simulink model "Task1_d"  (R2024b)
settings: Solver=VariableStepAuto  StartTime=0.0  StopTime=10.0  RelTol=1e-3
settings Model: Creator=max  LastModifiedBy=max

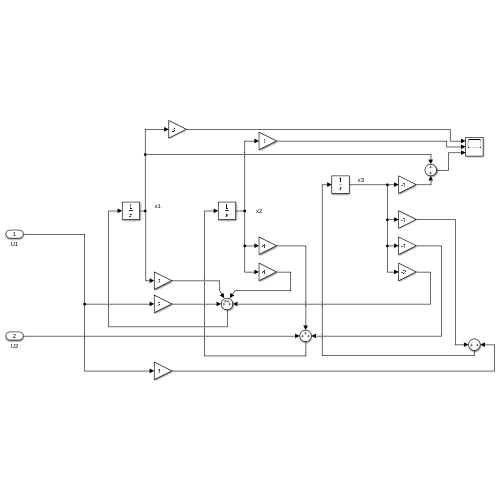
[thumbnail: Simulink's stored preview of the top-level diagram]
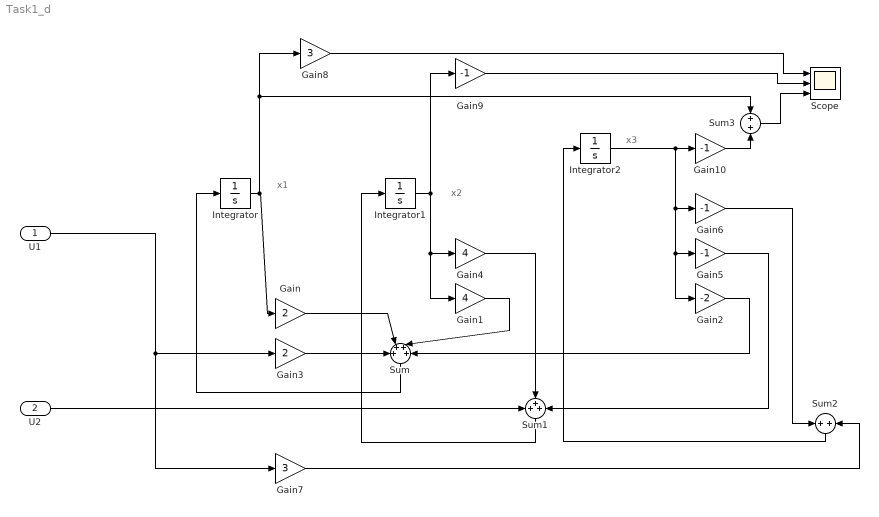
== system Task1_d ==
  note: x1
  note: x2
  note: x3
  U1 : Inport
  U2 : Inport  Port=2
  Gain : Gain  Gain=2
  Gain1 : Gain  Gain=4
  Gain{5..6,9..10} (4 alike) : Gain  Gain=-1
  Gain2 : Gain  Gain=-2
  Gain3 : Gain  Gain=2
  Gain4 : Gain  Gain=4
  Gain7 : Gain  Gain=3
  Gain8 : Gain  Gain=3
  Integrator : Integrator
  Integrator1 : Integrator
  Integrator2 : Integrator
  Scope : Scope  NumInputPorts=3
  Sum : Sum  Inputs=++++
  Sum1 : Sum  Inputs=+++
  Sum2 : Sum
  Sum3 : Sum
  wires:
  Integrator/1 -> Gain8/1, Sum3/1, Gain/1
  Gain/1 -> Sum/2
  Integrator1/1 -> Gain9/1, Gain4/1, Gain1/1
  Integrator2/1 -> Gain10/1, Gain6/1, Gain5/1, Gain2/1
  Gain1/1 -> Sum/3
  Gain2/1 -> Sum/4
  U1/1 -> Gain7/1, Gain3/1
  Gain3/1 -> Sum/1
  Sum/1 -> Integrator/1
  Gain4/1 -> Sum1/2
  Gain5/1 -> Sum1/3
  U2/1 -> Sum1/1
  Sum1/1 -> Integrator1/1
  Gain7/1 -> Sum2/2
  Sum2/1 -> Integrator2/1
  Gain6/1 -> Sum2/1
  Gain8/1 -> Scope/1
  Gain9/1 -> Scope/2
  Gain10/1 -> Sum3/2
  Sum3/1 -> Scope/3
